simulink model "mnist_softmax_figure"  (R2017b)
settings: Solver=FixedStepDiscrete  StartTime=0.0  StopTime=Inf  FixedStep=1  RelTol=1e-3
model workspace (MATLAB code in the model file):
  | BatchSize=100;
  | learningrate=0.05
undefined symbols (not defined in the file or in its folder): b_initial, W_initial
libraries: ad_blocks x12
settings Model: PauseTimes=2  SnapshotBufferSize=2  SnapshotInterval=1  Creator=percro2  LastModifiedBy=eruffaldi
settings CodeAppCC: StateflowObjectComments=on

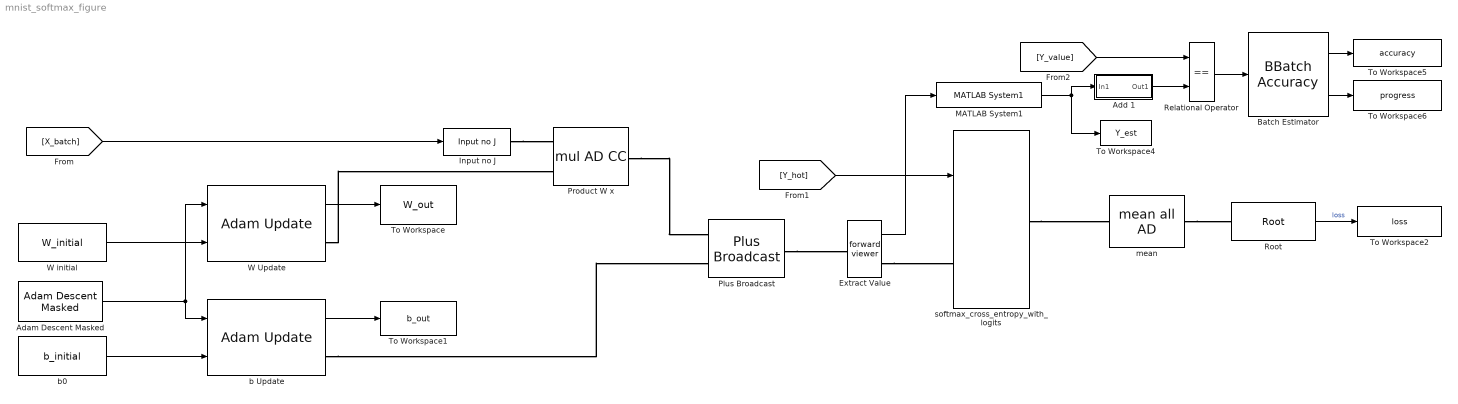
== system mnist_softmax_figure ==
  Adam Descent Masked : ad_blocks/Adam Descent Masked  learningrate=0.5  beta1=0.9  beta2=0.9999  epsilon=1e-8  adam=off
  Add 1 : Subsystem
  Batch Estimator : ad_blocks/BBatch Accuracy
  Extract Value : ad_blocks/forward viewer  SystemSampleTime=-1
  Input no J : ad_blocks/Input no J  SystemSampleTime=-1
  MATLAB System1 : ad_blocks/MATLAB System1  SimulateUsing=Interpreted execution
  Plus Broadcast : ad_blocks/Plus Broadcast
  Product W x : ad_blocks/mul AD CC
  Relational Operator : RelationalOperator  Operator===  OutDataTypeStr=boolean  RndMeth=Simplest
  Root : ad_blocks/Root  Description=Top level AD block: gets the incoming value, pushes the scalar 1 gradient  SystemSampleTime=-1
  To Workspace : ToWorkspace  VariableName=W_out  SaveFormat=Timeseries  SampleTime=-1
      settings: MaxDataPoints=1
  To Workspace1 : ToWorkspace  VariableName=b_out  SaveFormat=Timeseries  SampleTime=-1
      settings: MaxDataPoints=1
  To Workspace2 : ToWorkspace  VariableName=loss  SaveFormat=Timeseries  SampleTime=-1
      settings: MaxDataPoints=1
  To Workspace4 : ToWorkspace  VariableName=Y_est  SaveFormat=Timeseries  SampleTime=-1
      settings: MaxDataPoints=1
  To Workspace5 : ToWorkspace  VariableName=accuracy  SaveFormat=Timeseries  SampleTime=-1
      settings: MaxDataPoints=1
  To Workspace6 : ToWorkspace  VariableName=progress  SaveFormat=Timeseries  SampleTime=-1
      settings: MaxDataPoints=1
  W Update : ad_blocks/Adam Update
  W initial : Constant  Value=W_initial  OutDataTypeStr=single
  b Update : ad_blocks/Adam Update
  b0 : Constant  Value=b_initial  OutDataTypeStr=single
  mean : ad_blocks/mean all AD
  softmax_cross_entropy_with_logits : ad_blocks/softmax_cross_entropy_with_logits
  wires:
  Adam Descent Masked/1 -> b Update/1, W Update/1
  W initial/1 -> W Update/2
  W Update/1 -> To Workspace/1
  b Update/1 -> To Workspace1/1
  [Y_hot] -> softmax_cross_entropy_with_logits/1
  [Y_value] -> Relational Operator/1
  b0/1 -> b Update/2
  Extract Value/1 -> MATLAB System1/1
  Relational Operator/1 -> Batch Estimator/2
  Add 1/1(Out1) -> Relational Operator/2
  [X_batch] -> Input no J/1
  Root/1 -> To Workspace2/1  "loss"
  MATLAB System1/1 -> To Workspace4/1, Add 1/1(In1)
  Batch Estimator/1 -> To Workspace5/1
  Batch Estimator/2 -> To Workspace6/1
  connections:
  Input no J/RConn1 -- Product W x/LConn1
  W Update/RConn1 -- Product W x/LConn2
  mean/RConn1 -- Root/LConn1
  Product W x/RConn1 -- Plus Broadcast/LConn1
  b Update/RConn1 -- Plus Broadcast/LConn2
  Extract Value/RConn1 -- softmax_cross_entropy_with_logits/LConn1
  Plus Broadcast/RConn1 -- Extract Value/LConn1
  softmax_cross_entropy_with_logits/RConn1 -- mean/LConn1

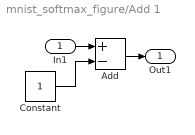
== system mnist_softmax_figure/Add 1 ==
  In1 : Inport
  Add : Sum  Inputs=+-
  Constant : Constant  OutDataTypeStr=Inherit: Inherit via back propagation
  Out1 : Outport
  wires:
  In1/1 -> Add/1
  Add/1 -> Out1/1
  Constant/1 -> Add/2
